simulink model "PlantaModelo3D"  (R2016a)
settings: Solver=VariableStepAuto  StartTime=0.0  StopTime=10  RelTol=1e-3
values from neighbouring files (symbols this model uses):
  s = tf('s')    [HinfPlantSeguroa.m]    (also in HinfPlanta.m)
undefined symbols (not defined in the file or in its folder): baseUnida, helice, Pieza2, PlantaUnida, RootGround, RootPart
libraries: mblibv1 x12, vrlib x1, simulink x1
settings Model: Creator=i95sa  LastModifiedBy=i95sa
settings GRTTargetCC: GeneratePreprocessorConditionals=Use local settings
settings SimMechanicsCC: VisOnUpdateDiagram=on  VisDuringSimulation=on  VisSampleTime=-1  AnimationDelay=0  LastVizWinPosition=[737 261 560 347]  CamPosition=[-4.10248;-9.8793;3.23212;]  CamTarget=[0.302765;0.111773;0.0269487;]  CamUpVector=[0.108641;0.25991;0.959502;]  CamHeight=0.475584  VisBackgroundColor=[0.9;0.9;0.95;]  DefaultBodyColor=[1;0;0;]

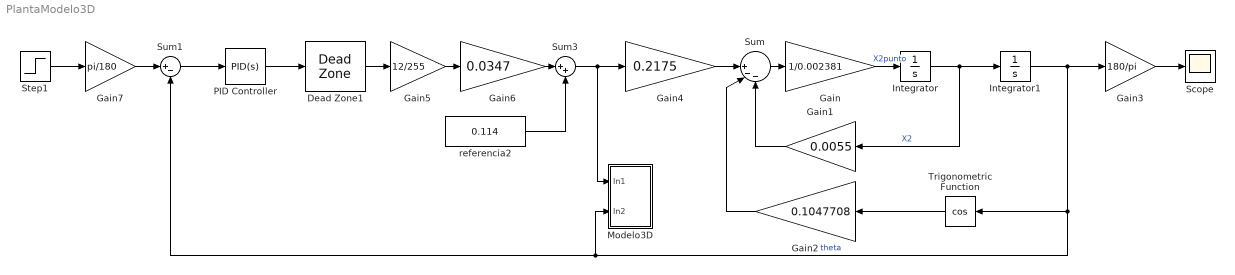
== system PlantaModelo3D ==
  Dead Zone1 : DeadZone  LowerValue=0  UpperValue=0  SaturateOnIntegerOverflow=on
  Gain : Gain  Gain=1/0.002381
  Gain1 : Gain  Gain=0.0055
  Gain2 : Gain  Gain=0.1047708
  Gain3 : Gain  Gain=180/pi
  Gain4 : Gain  Gain=0.2175
  Gain5 : Gain  Gain=12/255
  Gain6 : Gain  Gain=0.0347
  Gain7 : Gain  Gain=pi/180
  Integrator : Integrator
  Integrator1 : Integrator  InitialCondition=-0.65
  Modelo3D : Subsystem
  PID Controller : simulink/Continuous/PID Controller  Controller=PID  TimeDomain=Continuous-time  SampleTime=-1  IntegratorMethod=Forward Euler  FilterMethod=Forward Euler  Form=Parallel  UseFilter=on  ControllerParametersSource=internal  P=865.957655750314  I=1903.46906537449  D=97.9058017458791  N=1947.94278086494  InitialConditionSource=internal  InitialConditionForIntegrator=0  InitialConditionForFilter=0  ExternalReset=none  LimitOutput=on  UpperSaturationLimit=255  LowerSaturationLimit=0  LinearizeAsGain=off  AntiWindupMode=clamping  Kb=1  TrackingMode=off  Kt=1  PParamMin=[]  PParamMax=[]  IParamMin=[]  IParamMax=[]  DParamMin=[]  DParamMax=[]  NParamMin=[]  NParamMax=[]  KbParamMin=[]  KbParamMax=[]  KtParamMin=[]  KtParamMax=[]  POutMin=[]  POutMax=[]  IOutMin=[]  IOutMax=[]  DOutMin=[]  DOutMax=[]  NOutMin=[]  NOutMax=[]  KbOutMin=[]  KbOutMax=[]  KtOutMin=[]  KtOutMax=[]  IntegratorOutMin=[]  IntegratorOutMax=[]  FilterOutMin=[]  FilterOutMax=[]  SumOutMin=[]  SumOutMax=[]  SumI1OutMin=[]  SumI1OutMax=[]  SumI2OutMin=[]  SumI2OutMax=[]  SumI3OutMin=[]  SumI3OutMax=[]  SumDOutMin=[]  SumDOutMax=[]  SaturationOutMin=[]  SaturationOutMax=[]  IntegratorContinuousStateAttributes=''  IntegratorStateMustResolveToSignalObject=off  IntegratorRTWStateStorageClass=Auto  FilterContinuousStateAttributes=''  FilterStateMustResolveToSignalObject=off  FilterRTWStateStorageClass=Auto  DifferentiatorICPrevScaledInput=0  DifferentiatorOutMin=[]  DifferentiatorOutMax=[]
  Scope : Scope
  Step1 : Step  Time=0  After=20  SampleTime=0
  Sum : Sum  Inputs=||+--
  Sum1 : Sum  Inputs=|+-
  Sum3 : Sum  Inputs=|++
  Trigonometric Function : Trigonometry  Operator=cos
  referencia2 : Constant  Value=0.114
  wires:
  Sum/1 -> Gain/1
  Gain/1 -> Integrator/1  "X2punto"
  Integrator/1 -> Integrator1/1, Gain1/1  "X2"
  Trigonometric Function/1 -> Gain2/1
  Gain1/1 -> Sum/3
  Integrator1/1 -> Sum1/2, Modelo3D/2(In2), Trigonometric Function/1, Gain3/1  "theta"
  Gain2/1 -> Sum/2
  Gain4/1 -> Sum/1
  referencia2/1 -> Sum3/2
  Gain5/1 -> Gain6/1
  Gain6/1 -> Sum3/1
  Dead Zone1/1 -> Gain5/1
  Gain3/1 -> Scope/1
  Sum3/1 -> Modelo3D/1(In1), Gain4/1
  PID Controller/1 -> Dead Zone1/1
  Sum1/1 -> PID Controller/1
  Gain7/1 -> Sum1/1
  Step1/1 -> Gain7/1

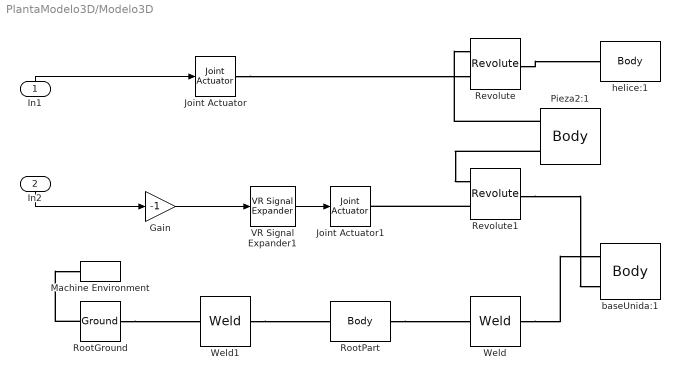
== system PlantaModelo3D/Modelo3D ==
  In1 : Inport
  In2 : Inport  Port=2
  Gain : Gain  Gain=-1
  Joint Actuator : mblibv1/Sensors &  Actuators/Joint Actuator  UpdateFromCAD=off  PhysicalDomain=Mechanical  PortType=blob  ActuationStyle=Force  AngleUnits=deg  ArcVelocityUnits=deg/s  ArcAccelerationUnits=deg/s^2  CoordPositionUnits=m  VelocityUnits=m/s  AccelerationUnits=m/s^2  ForceUnits=N  TorqueUnits=N-m  ActiveIO=on  Width=1  DialogClass=MechanicalActuatorBlock  Primitive=R1  ReferenceFrame=Absolute (World)
  Joint Actuator1 : mblibv1/Sensors &  Actuators/Joint Actuator  UpdateFromCAD=off  PhysicalDomain=Mechanical  PortType=blob  ActuationStyle=Motion  AngleUnits=rad  ArcVelocityUnits=rad/s  ArcAccelerationUnits=rad/s^2  CoordPositionUnits=m  VelocityUnits=m/s  AccelerationUnits=m/s^2  ForceUnits=N  TorqueUnits=N*m  ActiveIO=on  Width=3  DialogClass=MechanicalActuatorBlock  Primitive=R1  ReferenceFrame=Absolute (World)
  Machine Environment : mblibv1/Bodies/Machine Environment  PortType=env  PhysicalDomain=Mechanical  DialogTemplateClass=MECH.MachineEnvironment  SyncWhenCopied=off  Gravity=[0 -9.81 0]  GravityUnits=m/s^2  GravityAsSignal=off  Dimensionality=Auto-detect  AnalysisType=Forward dynamics  LinearAssemblyTolerance=1e-3  LinearAssemblyToleranceUnits=m  AngularAssemblyTolerance=1e-3  AngularAssemblyToleranceUnits=rad  ConstraintSolverType=Stabilizing  ConstraintRelTolerance=1e-4  ConstraintAbsTolerance=1e-4  UseRobustSingularityHandling=off  RedundancyAnalysisToleranceType=Automatically select tolerance  RedundancyAnalysisTolerance=1e-14  StatePerturbationType=Fixed  PerturbationSize=1e-5  VisualizeMachine=on  BodyVisualizationType=Use model default body geometries  BodyColorSelMode=Use model default  DefaultBodyColor=[1 0 0]
  Pieza2:1 : mblibv1/Bodies/Body  RConnTagsString=CS2|CS3  UpdateFromCAD=on  PMImportedID=Pieza2:1  DialogClass=MechanicalBodyBlock  Mass=0.0627209  MassUnits=kg  InertiaUnits=kg*m^2  Inertia=[9.17532e-05,5.485e-06,-0.000243037;5.485e-06,0.00080343,1.92748e-06;-0.000243037,1.92748e-06,0.000717235]  Shape=Cylinder  ShapeDims=[1 1]  ShapeUnits=m  ShapeUse=false  Density=1  DensityUnits=kg/m^3  DensityUse=false  GraphicsMode=GFXFILE  GraphicsFileName=Pieza2_ipt_8f5fd960.STL  BodyColorSelMode=COLORPALETTE  BodyColor=[1;1;1]  AttachedToCS=CS1  CG=Right$CG$[290.041 126.822 167.221]$WORLD$WORLD$mm$[0.951631 0 0.307243;0 1 0;-0.307243 0 0.951631]$3x3 Transform$rad$WORLD$false$Pieza2:1::CG(AUTOGEN)  WorkingFrames=Right$CS1$[256.927 125.661 -149.696]$WORLD$WORLD$mm$[0.951631 0 0.307243;0 1 0;-0.307243 0 0.951631]$3x3 Transform$rad$WORLD$false$Pieza2:1::CS1(AUTOGEN)#Right$CS2$[151.653 127.993 190.25]$WORLD$WORLD$mm$[1 0 0;0 1 0;0 0 1]$3x3 Transform$rad$WORLD$true$Pieza2:1:-:helice:1::Pieza2:1(AUTOGEN)#Right$CS3$[369.153 106.193 169.25]$WORLD$WORLD$mm$[1 0 0;0 1 0;0 0 1]$3x3 Transform$rad$WORLD$true$Pieza2:1:-:baseUnida:1::Pieza2:1(AUTOGEN)  CGPos=[290.041 126.822 167.221]  CGRot=[0.951631 0 0.307243;0 1 0;-0.307243 0 0.951631]  CS0Pos=[]  CS0Rot=[]  CS1Pos=[256.927 125.661 -149.696]  CS1Rot=[0.951631 0 0.307243;0 1 0;-0.307243 0 0.951631]  CS2Pos=[151.653 127.993 190.25]  CS2Rot=[1 0 0;0 1 0;0 0 1]  CS3Pos=[369.153 106.193 169.25]  CS3Rot=[1 0 0;0 1 0;0 0 1]  CS4Pos=[]  CS4Rot=[]  CS5Pos=[]  CS5Rot=[]  CS6Pos=[]  CS6Rot=[]  CS7Pos=[]  CS7Rot=[]  CS8Pos=[]  CS8Rot=[]  CS9Pos=[]  CS9Rot=[]  CS10Pos=[]  CS10Rot=[]  CS11Pos=[]  CS11Rot=[]  CS12Pos=[]  CS12Rot=[]  CS13Pos=[]  CS13Rot=[]  CS14Pos=[]  CS14Rot=[]  CS15Pos=[]  CS15Rot=[]  CS16Pos=[]  CS16Rot=[]  CS17Pos=[]  CS17Rot=[]  CS18Pos=[]  CS18Rot=[]  CS19Pos=[]  CS19Rot=[]  CS20Pos=[]  CS20Rot=[]
  Revolute : mblibv1/Joints/Revolute  LConnTagsString=__newl0|SA1  RConnTagsString=__newr0  UpdateFromCAD=on  PMImportedID=Pieza2:1:-:helice:1  NumSAPorts=1  CutJoint=off  MarkAsCut=off  Primitives=prismatic  PrimitiveProps=R1$World$[0,0,1]$revolute  DialogClass=JointBlock  R1Axis=[0,0,1]
  Revolute1 : mblibv1/Joints/Revolute  LConnTagsString=__newl0|SA1  RConnTagsString=__newr0  UpdateFromCAD=on  PMImportedID=Pieza2:1:-:baseUnida:1  NumSAPorts=1  CutJoint=off  MarkAsCut=off  Primitives=prismatic  PrimitiveProps=R1$World$[0,1,0]$revolute  DialogClass=JointBlock  R1Axis=[0,1,0]
  RootGround : mblibv1/Bodies/Ground  UpdateFromCAD=on  PMImportedID=RootGround  LeftPortType=env  RightPortType=workingframe  PhysicalDomain=Mechanical  DialogClass=GroundBlock  CoordPosition=[351.973,123.406,-64.4651]  CoordPositionUnits=mm  StateVectorMgrId=5  MachineId=[6 0]  ShowEnvPort=on  ParameterChecksum=[1759355927, 4156117003, 1752778195, 1594877027]  TopologyChecksum=[3851268166, 2355162070, 3809030896, 1746967506]
  RootPart : mblibv1/Bodies/Body  LConnTagsString=CS3  RConnTagsString=CS2  UpdateFromCAD=on  PMImportedID=PlantaUnida/RootPart  DialogClass=MechanicalBodyBlock  Mass=0  MassUnits=kg  InertiaUnits=kg*m^2  Inertia=[0,0,0;0,0,0;0,0,0]  Shape=Cylinder  ShapeDims=[1 1]  ShapeUnits=m  ShapeUse=false  Density=1  DensityUnits=kg/m^3  DensityUse=false  GraphicsMode=MACHINE_DEFAULT  BodyColorSelMode=MACHINE_DEFAULT  BodyColor=[1;0;0]  AttachedToCS=CS1  CG=Right$CG$[351.973 123.406 -64.4651]$WORLD$WORLD$mm$[1 0 0;0 1 0;0 0 1]$3x3 Transform$rad$WORLD$false$PlantaUnida/RootPart::CG(AUTOGEN)  WorkingFrames=Right$CS1$[0 0 0]$WORLD$WORLD$mm$[1 0 0;0 1 0;0 0 1]$3x3 Transform$rad$WORLD$false$PlantaUnida/RootPart::CS1(AUTOGEN)#Right$CS2$[354.172 123.292 -72.1537]$WORLD$WORLD$mm$[1 0 0;0 1 0;0 0 1]$3x3 Transform$rad$WORLD$true$PlantaUnida/RootPart:-:baseUnida:1::PlantaUnida/RootPart(AUTOGEN)#Left$CS3$[351.973 123.406 -64.4651]$WORLD$WORLD$mm$[1 0 0;0 1 0;0 0 1]$3x3 Transform$rad$WORLD$true$PlantaUnida/RootPart:-:RootGround::PlantaUnida/RootPart(AUTOGEN)  CGPos=[351.973 123.406 -64.4651]  CGRot=[1 0 0;0 1 0;0 0 1]  CS0Pos=[]  CS0Rot=[]  CS1Pos=[0 0 0]  CS1Rot=[1 0 0;0 1 0;0 0 1]  CS2Pos=[354.172 123.292 -72.1537]  CS2Rot=[1 0 0;0 1 0;0 0 1]  CS3Pos=[351.973 123.406 -64.4651]  CS3Rot=[1 0 0;0 1 0;0 0 1]  CS4Pos=[]  CS4Rot=[]  CS5Pos=[]  CS5Rot=[]  CS6Pos=[]  CS6Rot=[]  CS7Pos=[]  CS7Rot=[]  CS8Pos=[]  CS8Rot=[]  CS9Pos=[]  CS9Rot=[]  CS10Pos=[]  CS10Rot=[]  CS11Pos=[]  CS11Rot=[]  CS12Pos=[]  CS12Rot=[]  CS13Pos=[]  CS13Rot=[]  CS14Pos=[]  CS14Rot=[]  CS15Pos=[]  CS15Rot=[]  CS16Pos=[]  CS16Rot=[]  CS17Pos=[]  CS17Rot=[]  CS18Pos=[]  CS18Rot=[]  CS19Pos=[]  CS19Rot=[]  CS20Pos=[]  CS20Rot=[]
  VR Signal Expander1 : vrlib/VR Signal Expander  outwidth=3  outidx=[1 2 3]
  Weld : mblibv1/Joints/Weld  LConnTagsString=__newl0  RConnTagsString=__newr0  UpdateFromCAD=on  PMImportedID=PlantaUnida/RootPart:-:baseUnida:1  NumSAPorts=0  CutJoint=off  MarkAsCut=off  Primitives=weld  PrimitiveProps=W$WORLD$[0.57735,0.57735,0.57735]$weld  DialogClass=JointBlock  WAxis=[0.57735,0.57735,0.57735]
  Weld1 : mblibv1/Joints/Weld  LConnTagsString=__newl0  RConnTagsString=__newr0  UpdateFromCAD=on  PMImportedID=PlantaUnida/RootPart:-:RootGround  NumSAPorts=0  CutJoint=off  MarkAsCut=off  Primitives=weld  PrimitiveProps=W$WORLD$[0.57735,0.57735,0.57735]$weld  DialogClass=JointBlock  WAxis=[0.57735,0.57735,0.57735]
  baseUnida:1 : mblibv1/Bodies/Body  LConnTagsString=CS2|CS3  UpdateFromCAD=on  PMImportedID=baseUnida:1  DialogClass=MechanicalBodyBlock  Mass=1.96686  MassUnits=kg  InertiaUnits=kg*m^2  Inertia=[0.0189272,-0.000227924,-0.00177317;-0.000227924,0.0205312,0.00045363;-0.00177317,0.00045363,0.00567196]  Shape=Cylinder  ShapeDims=[1 1]  ShapeUnits=m  ShapeUse=false  Density=1  DensityUnits=kg/m^3  DensityUse=false  GraphicsMode=GFXFILE  GraphicsFileName=baseUnida_ipt_1244857d.STL  BodyColorSelMode=COLORPALETTE  BodyColor=[0.74902;0.74902;0.74902]  AttachedToCS=CS1  CG=Right$CG$[354.172 123.292 -72.1537]$WORLD$WORLD$mm$[1 0 0;0 1 0;0 0 1]$3x3 Transform$rad$WORLD$false$baseUnida:1::CG(AUTOGEN)  WorkingFrames=Right$CS1$[360.349 126.261 -168.75]$WORLD$WORLD$mm$[1 0 0;0 1 0;0 0 1]$3x3 Transform$rad$WORLD$false$baseUnida:1::CS1(AUTOGEN)#Left$CS2$[354.172 123.292 -72.1537]$WORLD$WORLD$mm$[1 0 0;0 1 0;0 0 1]$3x3 Transform$rad$WORLD$true$PlantaUnida/RootPart:-:baseUnida:1::baseUnida:1(AUTOGEN)#Left$CS3$[369.153 106.193 169.25]$WORLD$WORLD$mm$[1 0 0;0 1 0;0 0 1]$3x3 Transform$rad$WORLD$true$Pieza2:1:-:baseUnida:1::baseUnida:1(AUTOGEN)  CGPos=[354.172 123.292 -72.1537]  CGRot=[1 0 0;0 1 0;0 0 1]  CS0Pos=[]  CS0Rot=[]  CS1Pos=[360.349 126.261 -168.75]  CS1Rot=[1 0 0;0 1 0;0 0 1]  CS2Pos=[354.172 123.292 -72.1537]  CS2Rot=[1 0 0;0 1 0;0 0 1]  CS3Pos=[369.153 106.193 169.25]  CS3Rot=[1 0 0;0 1 0;0 0 1]  CS4Pos=[]  CS4Rot=[]  CS5Pos=[]  CS5Rot=[]  CS6Pos=[]  CS6Rot=[]  CS7Pos=[]  CS7Rot=[]  CS8Pos=[]  CS8Rot=[]  CS9Pos=[]  CS9Rot=[]  CS10Pos=[]  CS10Rot=[]  CS11Pos=[]  CS11Rot=[]  CS12Pos=[]  CS12Rot=[]  CS13Pos=[]  CS13Rot=[]  CS14Pos=[]  CS14Rot=[]  CS15Pos=[]  CS15Rot=[]  CS16Pos=[]  CS16Rot=[]  CS17Pos=[]  CS17Rot=[]  CS18Pos=[]  CS18Rot=[]  CS19Pos=[]  CS19Rot=[]  CS20Pos=[]  CS20Rot=[]
  helice:1 : mblibv1/Bodies/Body  LConnTagsString=CS2  UpdateFromCAD=on  PMImportedID=helice:1  DialogClass=MechanicalBodyBlock  Mass=0.00219538  MassUnits=kg  InertiaUnits=kg*m^2  Inertia=[1.26802e-06,1.27837e-06,2.82997e-11;1.27837e-06,1.40185e-06,-4.59181e-11;2.82997e-11,-4.59181e-11,2.64583e-06]  Shape=Cylinder  ShapeDims=[1 1]  ShapeUnits=m  ShapeUse=false  Density=1  DensityUnits=kg/m^3  DensityUse=false  GraphicsMode=GFXFILE  GraphicsFileName=helice_ipt_be61535d.STL  BodyColorSelMode=COLORPALETTE  BodyColor=[0.921569;0.921569;0.921569]  AttachedToCS=CS1  CG=Right$CG$[151.656 127.957 204.593]$WORLD$WORLD$mm$[-0.76863 -0.639693 0;0.639693 -0.76863 0;0 0 1]$3x3 Transform$rad$WORLD$false$helice:1::CG(AUTOGEN)  WorkingFrames=Right$CS1$[151.653 127.993 190.25]$WORLD$WORLD$mm$[-0.76863 -0.639693 0;0.639693 -0.76863 0;0 0 1]$3x3 Transform$rad$WORLD$false$helice:1::CS1(AUTOGEN)#Left$CS2$[151.653 127.993 190.25]$WORLD$WORLD$mm$[1 0 0;0 1 0;0 0 1]$3x3 Transform$rad$WORLD$true$Pieza2:1:-:helice:1::helice:1(AUTOGEN)  CGPos=[151.656 127.957 204.593]  CGRot=[-0.76863 -0.639693 0;0.639693 -0.76863 0;0 0 1]  CS0Pos=[]  CS0Rot=[]  CS1Pos=[151.653 127.993 190.25]  CS1Rot=[-0.76863 -0.639693 0;0.639693 -0.76863 0;0 0 1]  CS2Pos=[151.653 127.993 190.25]  CS2Rot=[1 0 0;0 1 0;0 0 1]  CS3Pos=[]  CS3Rot=[]  CS4Pos=[]  CS4Rot=[]  CS5Pos=[]  CS5Rot=[]  CS6Pos=[]  CS6Rot=[]  CS7Pos=[]  CS7Rot=[]  CS8Pos=[]  CS8Rot=[]  CS9Pos=[]  CS9Rot=[]  CS10Pos=[]  CS10Rot=[]  CS11Pos=[]  CS11Rot=[]  CS12Pos=[]  CS12Rot=[]  CS13Pos=[]  CS13Rot=[]  CS14Pos=[]  CS14Rot=[]  CS15Pos=[]  CS15Rot=[]  CS16Pos=[]  CS16Rot=[]  CS17Pos=[]  CS17Rot=[]  CS18Pos=[]  CS18Rot=[]  CS19Pos=[]  CS19Rot=[]  CS20Pos=[]  CS20Rot=[]
  wires:
  In1/1 -> Joint Actuator/1
  In2/1 -> Gain/1
  VR Signal Expander1/1 -> Joint Actuator1/1
  Gain/1 -> VR Signal Expander1/1
  connections:
  Joint Actuator/RConn1 -- Revolute/LConn2
  Revolute1/LConn2 -- Joint Actuator1/RConn1
  RootPart/RConn1 -- Weld/LConn1
  Pieza2:1/RConn2 -- Revolute1/LConn1
  Pieza2:1/RConn1 -- Revolute/LConn1
  Revolute1/RConn1 -- baseUnida:1/LConn2
  Weld/RConn1 -- baseUnida:1/LConn1
  Weld1/RConn1 -- RootPart/LConn1
  RootGround/RConn1 -- Weld1/LConn1
  Revolute/RConn1 -- helice:1/LConn1
  RootGround/LConn1 -- Machine Environment/RConn1
